simulink model "trim_Lagrangian_Model_Nonlinear"  (R2016a)
settings: Solver=VariableStepAuto  StartTime=0.0  StopTime=10.0  RelTol=1e-3
libraries: lib_Lagrangian_Model_Nonlinear x1
settings Model: Creator=ottoe  LastModifiedBy=ottoe

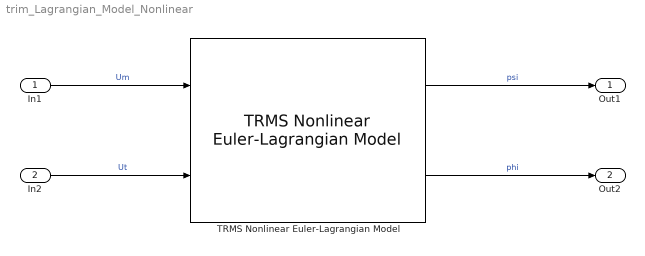
== system trim_Lagrangian_Model_Nonlinear ==
  In1 : Inport
  In2 : Inport  Port=2
  TRMS Nonlinear Euler-Lagrangian Model : lib_Lagrangian_Model_Nonlinear/TRMS Nonlinear Euler-Lagrangian Model  SystemSampleTime=-1
  Out1 : Outport
  Out2 : Outport  Port=2
  wires:
  In1/1 -> TRMS Nonlinear Euler-Lagrangian Model/1  "Um"
  In2/1 -> TRMS Nonlinear Euler-Lagrangian Model/2  "Ut"
  TRMS Nonlinear Euler-Lagrangian Model/1 -> Out1/1  "psi"
  TRMS Nonlinear Euler-Lagrangian Model/2 -> Out2/1  "phi"
